simulink model "a1ae2(1)"  (R2022a)
settings: Solver=VariableStepAuto  StartTime=0.0  StopTime=1000  RelTol=1e-3
settings Model: Creator=attit  LastModifiedBy=attit

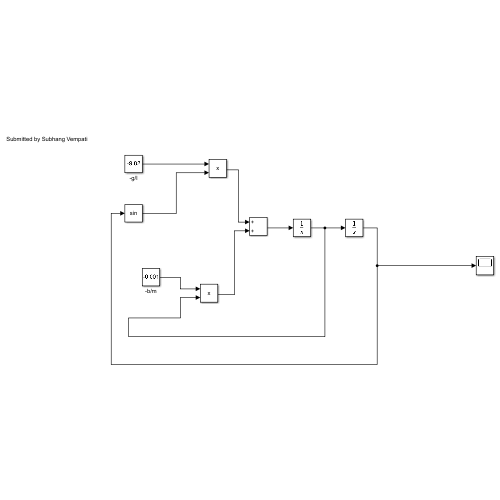
[thumbnail: Simulink's stored preview of the top-level diagram]
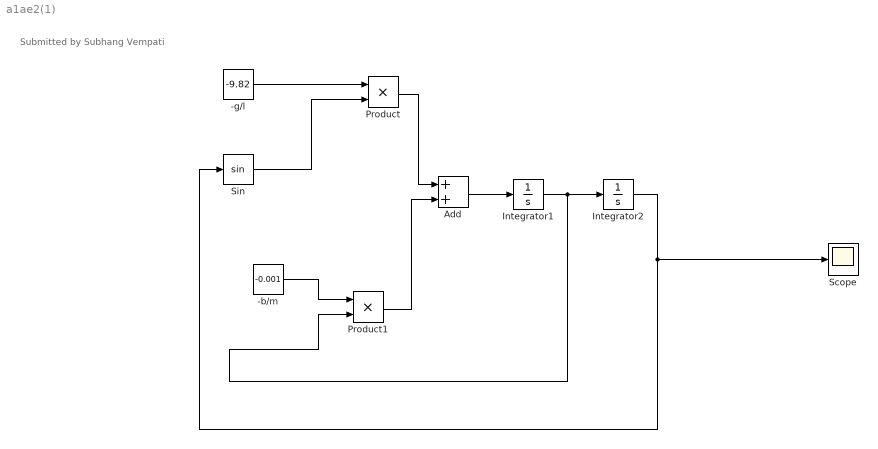
== system a1ae2(1) ==
  note: Submitted by Subhang Vempati
  -b/m : Constant  Value=-0.001
  -g/l : Constant  Value=-9.82
  Add : Sum
  Integrator1 : Integrator
  Integrator2 : Integrator  InitialCondition=pi/4
  Product : Product
  Product1 : Product
  Scope : Scope
  Sin : Trigonometry
  wires:
  -g/l/1 -> Product/1
  Sin/1 -> Product/2
  -b/m/1 -> Product1/1
  Product1/1 -> Add/2
  Product/1 -> Add/1
  Add/1 -> Integrator1/1
  Integrator2/1 -> Scope/1, Sin/1
  Integrator1/1 -> Product1/2, Integrator2/1
